simulink model "MARS"  (R2022a)
settings: Solver=VariableStepAuto  StartTime=0.0  StopTime=inf  RelTol=1e-3
model workspace (MAT data in the model file):
  T0 = -23.4
  h_trop = 7
  ingenuityParams : object (value not decoded)
symbols that are objects in the model workspace (value not decoded): ingenuityParams
undefined symbols (not defined in the file): body, collective1, collective2, duration, ingenuity, leg1, leg2, leg3, leg4, link_name, model_name, rotor1, rotor2, solarPanel, world_pose
libraries: fl_lib x35, robotgazebolib x31, nesl_utility x12, ee_lib x11, slpidlib x3, sharedtransform x2, simulink x1, shared6dof x1, aerolibwind2 x1
(part 2 of 3)

== system MARS/M.A.R.S./Force Components ==
  note: Subsystem
  In1 : Inport
  In2 : Inport  Port=2
  delta : Inport  Port=3
  epsilon : Inport  Port=4
  In5 : Inport  Port=5
  Components : Subsystem
  Product2 : Product
  Subsystem : Subsystem
  Out1 : Outport
  Out2 : Outport  Port=2
  Out3 : Outport  Port=3
  wires:
  Components/2(Out2) -> Subsystem/3(In3)
  Components/1(Out1) -> Subsystem/2(In2)
  Components/3(Out3) -> Subsystem/4(In4)
  In1/1 -> Product2/1
  Components/4(Out4) -> Subsystem/5(In5)
  Subsystem/2(Out2) -> Out2/1
  epsilon/1 -> Components/2(epsilon)
  Subsystem/1(Out1) -> Out1/1
  Product2/1 -> Subsystem/1(In1)
  Subsystem/3(Out3) -> Out3/1
  delta/1 -> Components/1(delta)
  In5/1 -> Subsystem/6(In6)
  In2/1 -> Product2/2

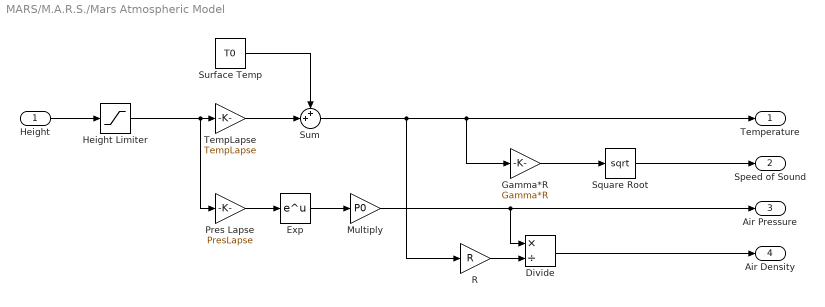
== system MARS/M.A.R.S./Mars Atmospheric Model ==
  Height : Inport
  Divide : Product  Inputs=*/
  Exp : Math
  Gamma*R : Gain  Gain=Gamma*R
  Height Limiter : Saturate  UpperLimit=height_lim  LowerLimit=0
  Multiply : Gain  Gain=P0
  Pres Lapse : Gain  Gain=PresLapse
  R : Gain  Gain=R
  Square Root : Sqrt
  Sum : Sum  Inputs=++|
  Surface Temp : Constant  Value=T0
  TempLapse : Gain  Gain=TempLapse
  Temperature : Outport  Unit=K  VectorParamsAs1DForOutWhenUnconnected=off
  Speed of Sound : Outport  Port=2  Unit=m/s  VectorParamsAs1DForOutWhenUnconnected=off
  Air Pressure : Outport  Port=3  Unit=Pa  VectorParamsAs1DForOutWhenUnconnected=off
  Air Density : Outport  Port=4  Unit=kg/m^3  VectorParamsAs1DForOutWhenUnconnected=off
  wires:
  TempLapse/1 -> Sum/2
  Surface Temp/1 -> Sum/1
  Sum/1 -> Gamma*R/1, Temperature/1, R/1
  Pres Lapse/1 -> Exp/1
  Exp/1 -> Multiply/1
  Multiply/1 -> Divide/1, Air Pressure/1
  Height/1 -> Height Limiter/1
  Height Limiter/1 -> Pres Lapse/1, TempLapse/1
  Gamma*R/1 -> Square Root/1
  Square Root/1 -> Speed of Sound/1
  R/1 -> Divide/2
  Divide/1 -> Air Density/1

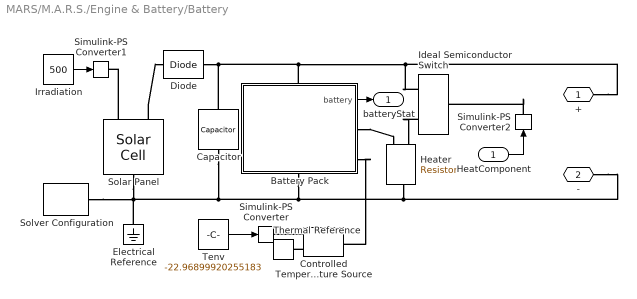
== system MARS/M.A.R.S./Engine & Battery/Battery ==
  HeatComponent : Inport
  Battery Pack : Subsystem  Variant=on  VariantControlMode=label  LabelModeActiveChoice=Detailed Battery Pack
      settings: PortSchema="{\"entries\":[{\"content\":{\"sides\":[{\"content\":{\"connectorIds\":[]},\"type\":\"ConnectorPlacement.EquallySpacedRectSide\",\"uuid\":\"b9ff85f5-5d37-4551-b274-b4f400e31e90\"},{\"content\":{\"connectorIds\":[\"Out1\",\"RConn1\",\"RConn2\"],\"side\":\"RIGHT\"},\"type\":\"ConnectorPlacement.EquallySpacedRectSide\",\"uuid\":\"9895ebaf-077a-447d-9f12-67b2d221f552\"},{\"content\":{\"connectorIds\":[\"LConn1\"],\"side\":\"TOP\"},\"type\":\"ConnectorPlacement.EquallySpacedRectSide\",\"uuid\":\"1c6b4d28-0fee-40d3-aeb3-8529f8417079\"},{\"content\":{\"connectorIds\":[\"RConn3\"],\"side\":\"BOTTOM\"},\"type\":\"ConnectorPlacement.EquallySpacedRectSide\",\"uuid\":\"bb08ee4d-4e3f-4517-9dbc-020c674c7490\"}]},\"type\":\"ConnectorPlacement.EquallySpacedConnector\",\"uuid\":\"d782096a-eb61-452d-945f-a15e6ccd7694\"}],\"packageUris\":[\"http://schema.mathworks.com/mf0/Connector/R2020b\"],\"version\":\"1.0\"}"
  Capacitor : fl_lib/Electrical/Electrical Elements/Capacitor  c=1e-6 F  r=1e-3 Ohm  g=0 1/Ohm  i_specify=off  i_priority=None  i=0 A  i_nominal_specify=off  i_nominal_unit=A  i_nominal_value=1  v_specify=off  v_priority=None  v=0 V  v_nominal_specify=off  v_nominal_unit=V  v_nominal_value=1  vc_specify=on  vc_priority=High  vc=24 V  vc_nominal_specify=off  vc_nominal_unit=V  vc_nominal_value=1
      settings: SourceProductBaseCode=PW,SS,VE  LogSimulationData=on
  Controlled Temperature Source : fl_lib/Thermal/Thermal Sources/Controlled Temperature Source
      settings: SourceProductBaseCode=PW,SS,VE
  Diode : fl_lib/Electrical/Electrical Elements/Diode  Vf=0.6 V  Ron=0.3 Ohm  Goff=1e-8 1/Ohm  i_specify=off  i_priority=None  i=0 A  i_nominal_specify=off  i_nominal_unit=A  i_nominal_value=1  v_specify=off  v_priority=None  v=0 V  v_nominal_specify=off  v_nominal_unit=V  v_nominal_value=1
      settings: SourceProductBaseCode=PW,SS,VE  LogSimulationData=on
  Electrical Reference : fl_lib/Electrical/Electrical Elements/Electrical Reference
      settings: SourceProductBaseCode=PW,SS,VE
  Heater : ee_lib/Passive/Resistor  R=2 Ohm  enable_R_tol=0  R_tol=5  tol_distribution=1  nSigma=4  enable_operating_limits=0  operating_limit_action=2  max_working_voltage=100 V  power_rating=1 W  enable_faults=0  fault_action=1  R_faulted=inf Ohm  enable_temporal_fault=0  t_fault=1 s  enable_behavioral_fault=0  max_permissible_current=1 A  t_fail_on_current=1 s  noise_mode=0  sample_time=1e-3 s  repeatability=1  auto_seed=3499211588  user_seed=0  Tdevice=25 degC  power_derating_T1=70 degC  power_derating_T2=155 degC  operating_temperature_range_vec=[-50, 150] degC  alpha=3.93e-3 1/K  Tmeas=25 degC  thermal_mass=ingenuityParams.heater.thermalMass J/K  temperature_specify=on  temperature_priority=None  temperature=ingenuityParams.battery.cell.T_init degC  temperature_nominal_specify=off  temperature_nominal_unit=K  temperature_nominal_value=1
      settings: LogSimulationData=on  InternalSimscapePortConfiguration="{\"Bottom\":[],\"Left\":[{\"id\":\"p\",\"label\":\"+\",\"type\":\"foundation.electrical.electrical\"},{\"id\":\"H\",\"label\":\"H\",\"type\":\"foundation.thermal.thermal\"}],\"Right\":[{\"id\":\"n\",\"label\":\"-\",\"type\":\"foundation.electrical.electrical\"}],\"Top\":[]}"
  Ideal Semiconductor Switch : ee_lib/Semiconductors & Converters/Ideal Semiconductor Switch  Ron=0.001 Ohm  Goff=1e-6 1/Ohm  Vth=0.5 V  diode_param=1  diode_Vf=0.8 V  diode_Ron=0.001 Ohm  diode_Goff=1e-5 1/Ohm  diode_C=50e-9 F  diode_iRM=-235 A  diode_iF=300 A  diode_idot=-50 A/us  diode_trr_param=1  diode_trr_factor=3  diode_trr=15 us  diode_Qrr=1500 s*uA
      settings: SourceProductBaseCode=PS  LogSimulationData=on
  Irradiation : Constant  Value=500
  Simulink-PS Converter : nesl_utility/Simulink-PS Converter  PhysicalDomain=network_engine_domain  SubClassName=ps_input  LeftPortType=input  RightPortType=output  PseudoPeriodic=off  Frequencies=[]  NoiseDistribution=none  NoiseParameters=[]  Unit=degC  AffineConversion=on  FilteringAndDerivatives=provide  SimscapeFilterOrder=1  InputFilterTimeConstant=0.001  UdotUserProvided=0
      settings: SourceProductBaseCode=SS,PW,VE
  Simulink-PS Converter1 : nesl_utility/Simulink-PS Converter  PhysicalDomain=network_engine_domain  SubClassName=ps_input  LeftPortType=input  RightPortType=output  PseudoPeriodic=off  Frequencies=[]  NoiseDistribution=none  NoiseParameters=[]  Unit=W/m^2  AffineConversion=off  FilteringAndDerivatives=provide  SimscapeFilterOrder=1  InputFilterTimeConstant=0.001  UdotUserProvided=0
      settings: SourceProductBaseCode=SS,PW,VE
  Simulink-PS Converter2 : nesl_utility/Simulink-PS Converter  PhysicalDomain=network_engine_domain  SubClassName=ps_input  LeftPortType=input  RightPortType=output  PseudoPeriodic=off  Frequencies=[]  NoiseDistribution=none  NoiseParameters=[]  Unit=V  AffineConversion=off  FilteringAndDerivatives=provide  SimscapeFilterOrder=1  InputFilterTimeConstant=0.001  UdotUserProvided=0
      settings: SourceProductBaseCode=SS,PW,VE
  Solar Panel : ee_lib/Sources/Solar Cell  prm=1  Isc=ingenuityParams.solarcells.Isc A  Voc=ingenuityParams.solarcells.Voc V  Is=1e-6 A  Is2=0 A  Iph=7.34 A  Ir0=ingenuityParams.solarcells.Ir0 W/m^2  ec=ingenuityParams.solarcells.qualFactor  N2=2  Rs=ingenuityParams.solarcells.Rs Ohm  Rp=inf Ohm  N_series=ingenuityParams.solarcells.Nseries  N_parallel=ingenuityParams.solarcells.Nparallel  TIPH1=0 1/K  EG=1.11 eV  TXIS1=3  TXIS2=3  TRS1=0  TRP1=0  Tmeas=25 degC  TFIXED=25 degC  thermal_mass=100 J/K  initial_temperature=25 degC
      settings: SourceProductBaseCode=PS  LogSimulationData=on
  Solver Configuration : nesl_utility/Solver Configuration  PhysicalDomain=network_engine_domain  SubClassName=solver  LeftPortType=input  RightPortType=generic  Tones=[]  Harmonics=[]  SimulateNoise=off  Profile=off  UseLocalSampling=off  EnableSwitchedLinearOptims=on  FrequencyDomain=off  UseCCode=off  RelTol=0.001  AbsTol=1e-06  MinStep=1e-09  ToWorkspace=off  RevertToSquareIcSolve=off  NumHomotopyIterations=100  PhasorMode=off  PhasorModeNumHarmonics=1  IndexReductionMethod=DerivativeReplacement  DoDC=off  ResidualTolerance=1e-09  UseLocalSolver=off  LocalSolverChoice=NE_BACKWARD_EULER_ADVANCER  LocalSolverSampleTime=0.001  DoFixedCost=off  MaxNonlinIter=3  MaxModeIter=2  ComputeImpulses=off  ImpulseIterations=2  LinearAlgebra=auto  LinearAlgebraNumThread=0  EquationFormulation=NE_TIME_EF  DelaysMemoryBudget=1024  AutomaticFiltering=on  FilteringTimeConstant=0.001  PartitionStorageMethod=AS_NEEDED  PartitionMemoryBudget=1024  PartitionMethod=ROBUST
      settings: SourceProductBaseCode=SS,PW,VE
  Tenv : Constant  Value=-22.96899920255183
  Thermal Reference : fl_lib/Thermal/Thermal Elements/Thermal Reference
      settings: SourceProductBaseCode=PW,SS,VE
  + : PMIOPort  Side=Left
  - : PMIOPort  Port=2  Side=Left
  batteryStat : Outport
  wires:
  Tenv/1 -> Simulink-PS Converter/1
  Battery Pack/1(battery) -> batteryStat/1
  HeatComponent/1 -> Simulink-PS Converter2/1
  Irradiation/1 -> Simulink-PS Converter1/1
  connections:
  Solar Panel/LConn2 -- Diode/LConn1
  Capacitor/LConn1 -- +/RConn1 -- Ideal Semiconductor Switch/RConn1 -- Battery Pack/LConn1 -- Diode/RConn1
  Controlled Temperature Source/RConn1 -- Simulink-PS Converter/RConn1
  Heater/RConn1 -- -/RConn1 -- Solver Configuration/RConn1 -- Electrical Reference/LConn1 -- Solar Panel/RConn1 -- Capacitor/RConn1 -- Battery Pack/RConn3
  Simulink-PS Converter2/RConn1 -- Ideal Semiconductor Switch/LConn1
  Ideal Semiconductor Switch/RConn2 -- Heater/LConn1
  Controlled Temperature Source/RConn2 -- Thermal Reference/LConn1
  Solar Panel/LConn1 -- Simulink-PS Converter1/RConn1
  Battery Pack/RConn2 -- Controlled Temperature Source/LConn1
  Battery Pack/RConn1 -- Heater/LConn2

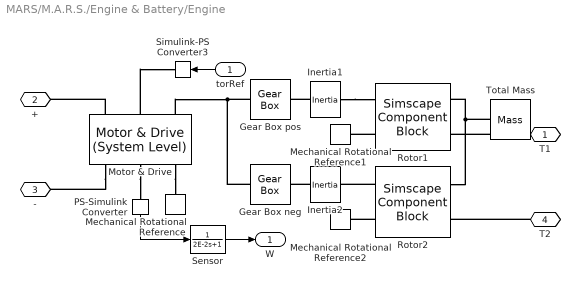
== system MARS/M.A.R.S./Engine & Battery/Engine ==
  torRef : Inport
  Gear Box neg : fl_lib/Mechanical/Mechanisms/Gear Box  ratio=-1*ingenuityParams.gearbox.ratio  t_in_specify=off  t_in_priority=None  t_in=0 N*m  t_in_nominal_specify=off  t_in_nominal_unit=N*m  t_in_nominal_value=1  t_out_specify=off  t_out_priority=None  t_out=0 N*m  t_out_nominal_specify=off  t_out_nominal_unit=N*m  t_out_nominal_value=1
      settings: SourceProductBaseCode=PW,SS,VE  LogSimulationData=on
  Gear Box pos : fl_lib/Mechanical/Mechanisms/Gear Box  ratio=ingenuityParams.gearbox.ratio  t_in_specify=off  t_in_priority=None  t_in=0 N*m  t_in_nominal_specify=off  t_in_nominal_unit=N*m  t_in_nominal_value=1  t_out_specify=off  t_out_priority=None  t_out=0 N*m  t_out_nominal_specify=off  t_out_nominal_unit=N*m  t_out_nominal_value=1
      settings: SourceProductBaseCode=PW,SS,VE  LogSimulationData=on
  Inertia1 : fl_lib/Mechanical/Rotational Elements/Inertia  inertia=ingenuityParams.propeller.inertia kg*m^2  num_ports=foundation.enum.numPorts2.two  w_specify=off  w_priority=High  w=0 rad/s  w_nominal_specify=off  w_nominal_unit=rad/s  w_nominal_value=1  t_specify=off  t_priority=None  t=0 N*m  t_nominal_specify=off  t_nominal_unit=N*m  t_nominal_value=1
      settings: SourceProductBaseCode=PW,SS,VE  LogSimulationData=on  InternalSimscapePortConfiguration="{\"Bottom\":[],\"Left\":[{\"id\":\"I\",\"label\":\"\",\"type\":\"foundation.mechanical.rotational.rotational\"}],\"Right\":[{\"id\":\"J\",\"label\":\"\",\"type\":\"foundation.mechanical.rotational.rotational\"}],\"Top\":[]}"
  Inertia2 : fl_lib/Mechanical/Rotational Elements/Inertia  inertia=ingenuityParams.propeller.inertia kg*m^2  num_ports=foundation.enum.numPorts2.two  w_specify=off  w_priority=High  w=0 rad/s  w_nominal_specify=off  w_nominal_unit=rad/s  w_nominal_value=1  t_specify=off  t_priority=None  t=0 N*m  t_nominal_specify=off  t_nominal_unit=N*m  t_nominal_value=1
      settings: SourceProductBaseCode=PW,SS,VE  LogSimulationData=on  InternalSimscapePortConfiguration="{\"Bottom\":[],\"Left\":[{\"id\":\"I\",\"label\":\"\",\"type\":\"foundation.mechanical.rotational.rotational\"}],\"Right\":[{\"id\":\"J\",\"label\":\"\",\"type\":\"foundation.mechanical.rotational.rotational\"}],\"Top\":[]}"
  Mechanical Rotational Reference : fl_lib/Mechanical/Rotational Elements/Mechanical Rotational Reference
      settings: SourceProductBaseCode=PW,SS,VE
  Mechanical Rotational Reference1 : fl_lib/Mechanical/Rotational Elements/Mechanical Rotational Reference
      settings: SourceProductBaseCode=PW,SS,VE
  Mechanical Rotational Reference2 : fl_lib/Mechanical/Rotational Elements/Mechanical Rotational Reference
      settings: SourceProductBaseCode=PW,SS,VE
  Motor & Drive : ee_lib/Electromechanical/Motor & Drive (System Level)  torque_speed_param=ee.enum.electromech.envelope.torque_power  overtorque_param=ee.enum.electromech.overtorque.no  T_t=[.09, .08, .07, 0] N*m  T_t_intermittent=[.36, .32, .28, 0] N*m  T_t_2D=[.09, .09, .09; .08, .08, .08; .07, .07, .07; 0, 0, 0] N*m  T_t_intermittent_2D=[.36, .36, .36; .32, .32, .32; .28, .28, .28; 0, 0, 0] N*m  w_t=[0, 3750, 7500, 8000] rpm  vdc_t=[6, 12, 24] V  torque_max=ingenuityParams.motordrive.torMax N*m  power_max=ingenuityParams.motordrive.powMax W  torque_max_intermittent=0.4 N*m  power_max_intermittent=120 W  time_overtorque=30 s  time_recover=60 s  Tc=ingenuityParams.motordrive.Tc s  losses_param=1  eff=ingenuityParams.motordrive.effRated  w_eff=ingenuityParams.motordrive.wRated rpm  T_eff=ingenuityParams.motordrive.torRated N*m  Piron=ingenuityParams.motordrive.ironLoss W  Pbase=ingenuityParams.motordrive.fixedLoss W  w_eff_vec=[-8000, -4000, 0, 4000, 8000] rpm  T_eff_vec=[0, .03, .06, .09] N*m  v_eff_vec=[100, 250, 400] V  losses_mat=[1.49, 1.67, 2.21, 3.1; .42, .69, 1.14, 2.03; .06, .24, .78, 1.68; .42, .69, 1.14, 2.03; 1.49, 1.67, 2.21, 3.1] W  efficiency_mat=[95, 95, 95, 95; 95, 95, 95, 95; 95, 95, 95, 95; 95, 95, 95, 95; 95, 95, 95, 95]  losses_mat_3D=ones(5, 4, 3) W  efficiency_mat_3D=95 * ones(5, 4, 3)  Res=ingenuityParams.motordrive.supplyRes Ohm  enable_fault=simscape.enum.onoff.off  fault_condition=1  fault_threshold=0.5  J=0 kg*m^2  lam=0 N*m/(rad/s)  speed0=0 rpm  faulted_specify=off  faulted_priority=None  faulted=0  faulted_nominal_specify=off  faulted_nominal_unit=1  faulted_nominal_value=1  torqueLimitContinuous_specify=off  torqueLimitContinuous_priority=None  torqueLimitContinuous=0 N*m  torqueLimitContinuous_nominal_specify=off  torqueLimitContinuous_nominal_unit=N*m  torqueLimitContinuous_nominal_value=1  alpha=3.93e-3 1/K  Tmeas=25 degC  Tmeas2=125 degC  losses_mat_T2=[1.49, 1.74, 2.49, 3.74; .42, .67, 1.42, 2.67; .06, .31, 1.06, 2.31; .42, .67, 1.42, 2.67; 1.49, 1.74, 2.49, 3.74] W  efficiency_mat_T2=[95, 95, 95, 95; 95, 95, 95, 95; 95, 95, 95, 95; 95, 95, 95, 95; 95, 95, 95, 95]  losses_mat_3D_T2=ones(5, 4, 3) W  efficiency_mat_3D_T2=95 * ones(5, 4, 3)  thermal_mass=100 J/K  initial_temperature=25 degC
      settings: SourceProductBaseCode=PS  LogSimulationData=on
  PS-Simulink Converter : nesl_utility/PS-Simulink Converter  PhysicalDomain=network_engine_domain  SubClassName=ps_output  LeftPortType=input  RightPortType=output  PseudoPeriodic=off  Frequencies=[]  VectorFormat=1-D array  Unit=rad/s  AffineConversion=off
      settings: SourceProductBaseCode=SS,PW,VE
  Rotor1 : SimscapeComponentBlock  SourceFile=simple_rotor  ComponentPath=simple_rotor  ComponentVariants="[\"simple_rotor\"]"  ComponentVariantNames="[\"simple_rotor\"]"  ClassName=simple_rotor  SchemaVersion=1  rot_dir=simscape.enum.posneg.positive  D=ingenuityParams.propeller.diameter m  J_TLU=ingenuityParams.propeller.Jvec  k_thrust_TLU=ingenuityParams.propeller.kTvec  k_power_TLU=ingenuityParams.propeller.kPvec  interp_method=simscape.enum.interpolation.smooth  extrap_method=simscape.enum.extrapolation.linear  density=ingenuityParams.environment.atmDensity kg/m^3  n_thr=1e-2 Hz  w_specify=on  w_priority=None  w=0 rpm  w_nominal_specify=off  w_nominal_unit=rad/s  w_nominal_value=1  Q_specify=off  Q_priority=None  Q=0 N*m  Q_nominal_specify=off  Q_nominal_unit=N*m  Q_nominal_value=1
      settings: CopyFcn=simscape.engine.sli.internal.componentblockcallback(gcbh,'COPY')  PreCopyFcn=simscape.engine.sli.internal.componentblockcallback(gcbh,'PRECOPY')  PreDeleteFcn=simscape.engine.sli.internal.componentblockcallback(gcbh,'PREDELETE')  InternalSimscapePortConfiguration="{\"Bottom\":[],\"Left\":[{\"id\":\"R\",\"label\":\"R\",\"type\":\"foundation.mechanical.rotational.rotational\"},{\"id\":\"C\",\"label\":\"C\",\"type\":\"foundation.mechanical.rotational.rotational\"}],\"Right\":[{\"id\":\"V\",\"label\":\"V\",\"type\":\"foundation.mechanical.translational.translational\"},{\"id\":\"T\",\"label\":\"T\",\"type\":\"output\"}],\"Top\":[]}"
      mask Type: Simple Rotor
  Rotor2 : SimscapeComponentBlock  SourceFile=simple_rotor  ComponentPath=simple_rotor  ComponentVariants="[\"simple_rotor\"]"  ComponentVariantNames="[\"simple_rotor\"]"  ClassName=simple_rotor  SchemaVersion=1  rot_dir=simscape.enum.posneg.positive  D=ingenuityParams.propeller.diameter m  J_TLU=ingenuityParams.propeller.Jvec  k_thrust_TLU=ingenuityParams.propeller.kTvec  k_power_TLU=ingenuityParams.propeller.kPvec  interp_method=simscape.enum.interpolation.smooth  extrap_method=simscape.enum.extrapolation.linear  density=ingenuityParams.environment.atmDensity kg/m^3  n_thr=1e-2 Hz  w_specify=on  w_priority=None  w=0 rpm  w_nominal_specify=off  w_nominal_unit=rad/s  w_nominal_value=1  Q_specify=off  Q_priority=None  Q=0 N*m  Q_nominal_specify=off  Q_nominal_unit=N*m  Q_nominal_value=1
      settings: CopyFcn=simscape.engine.sli.internal.componentblockcallback(gcbh,'COPY')  PreCopyFcn=simscape.engine.sli.internal.componentblockcallback(gcbh,'PRECOPY')  PreDeleteFcn=simscape.engine.sli.internal.componentblockcallback(gcbh,'PREDELETE')  InternalSimscapePortConfiguration="{\"Bottom\":[],\"Left\":[{\"id\":\"R\",\"label\":\"R\",\"type\":\"foundation.mechanical.rotational.rotational\"},{\"id\":\"C\",\"label\":\"C\",\"type\":\"foundation.mechanical.rotational.rotational\"}],\"Right\":[{\"id\":\"V\",\"label\":\"V\",\"type\":\"foundation.mechanical.translational.translational\"},{\"id\":\"T\",\"label\":\"T\",\"type\":\"output\"}],\"Top\":[]}"
      mask Type: Simple Rotor
  Sensor : TransferFcn  Denominator=[2E-2 1]
  Simulink-PS Converter3 : nesl_utility/Simulink-PS Converter  PhysicalDomain=network_engine_domain  SubClassName=ps_input  LeftPortType=input  RightPortType=output  PseudoPeriodic=off  Frequencies=[]  NoiseDistribution=none  NoiseParameters=[]  Unit=N*m  AffineConversion=off  FilteringAndDerivatives=provide  SimscapeFilterOrder=1  InputFilterTimeConstant=0.001  UdotUserProvided=0
      settings: SourceProductBaseCode=SS,PW,VE
  Total Mass : fl_lib/Mechanical/Translational Elements/Mass  mass=ingenuityParams.mechanical.totalMassExceptBatteries + ingenuityParams.battery.numCells*ingenuityParams.battery.cell.mass kg  num_ports=foundation.enum.numPorts2.one  v_specify=off  v_priority=High  v=0 m/s  v_nominal_specify=off  v_nominal_unit=m/s  v_nominal_value=1  f_specify=off  f_priority=None  f=0 N  f_nominal_specify=off  f_nominal_unit=N  f_nominal_value=1
      settings: SourceProductBaseCode=PW,SS,VE  LogSimulationData=on
  T1 : PMIOPort  Side=Right
  + : PMIOPort  Port=2  Side=Left
  - : PMIOPort  Port=3  Side=Left
  T2 : PMIOPort  Port=4  Side=Right
  W : Outport
  wires:
  torRef/1 -> Simulink-PS Converter3/1
  Sensor/1 -> W/1
  PS-Simulink Converter/1 -> Sensor/1
  connections:
  Inertia1/RConn1 -- Gear Box pos/RConn1
  Inertia2/RConn1 -- Gear Box neg/RConn1
  T1/RConn1 -- Rotor1/RConn2
  Inertia1/LConn1 -- Rotor1/LConn1
  Motor & Drive/LConn1 -- +/RConn1
  Rotor1/LConn2 -- Mechanical Rotational Reference1/LConn1
  Motor & Drive/RConn2 -- PS-Simulink Converter/LConn1
  Motor & Drive/LConn2 -- Simulink-PS Converter3/RConn1
  T2/RConn1 -- Rotor2/RConn2
  Gear Box pos/LConn1 -- Motor & Drive/LConn3 -- Gear Box neg/LConn1
  Motor & Drive/RConn1 -- -/RConn1
  Motor & Drive/RConn3 -- Mechanical Rotational Reference/LConn1
  Rotor2/LConn1 -- Inertia2/LConn1
  Total Mass/LConn1 -- Rotor2/RConn1 -- Rotor1/RConn1
  Rotor2/LConn2 -- Mechanical Rotational Reference2/LConn1

== system MARS/M.A.R.S./Force Components/Components ==
  delta : Inport
  epsilon : Inport  Port=2
  Cos : Trigonometry  Operator=cos
  Cos1 : Trigonometry  Operator=cos
  Sin : Trigonometry
  Sin1 : Trigonometry
  Out1 : Outport
  Out2 : Outport  Port=2
  Out3 : Outport  Port=3
  Out4 : Outport  Port=4
  wires:
  delta/1 -> Cos/1, Sin/1
  Sin1/1 -> Out4/1
  Cos/1 -> Out1/1
  Cos1/1 -> Out2/1
  Sin/1 -> Out3/1
  epsilon/1 -> Cos1/1, Sin1/1

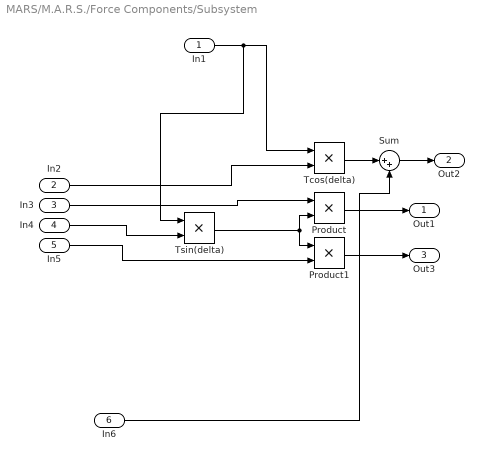
== system MARS/M.A.R.S./Force Components/Subsystem ==
  In1 : Inport
  In2 : Inport  Port=2
  In3 : Inport  Port=3
  In4 : Inport  Port=4
  In5 : Inport  Port=5
  In6 : Inport  Port=6
  Product : Product
  Product1 : Product
  Sum : Sum  Inputs=|++
  Tcos(delta) : Product
  Tsin(delta) : Product
  Out1 : Outport
  Out2 : Outport  Port=2
  Out3 : Outport  Port=3
  wires:
  In6/1 -> Sum/2
  Product1/1 -> Out3/1
  In1/1 -> Tsin(delta)/1, Tcos(delta)/1
  Tsin(delta)/1 -> Product/2, Product1/1
  In4/1 -> Tsin(delta)/2
  Tcos(delta)/1 -> Sum/1
  In5/1 -> Product1/2
  Product/1 -> Out1/1
  In2/1 -> Tcos(delta)/2
  In3/1 -> Product/1
  Sum/1 -> Out2/1

== system MARS/M.A.R.S./Engine & Battery/Battery/Battery Pack ==
  Detailed Battery Pack : Subsystem  VariantControl=Detailed Battery Pack
      settings: PortSchema="{\"entries\":[{\"content\":{\"sides\":[{\"content\":{\"connectorIds\":[]},\"type\":\"ConnectorPlacement.EquallySpacedRectSide\",\"uuid\":\"ac491242-3df9-473d-beed-1a2139a6c6bd\"},{\"content\":{\"connectorIds\":[\"Out1\",\"RConn1\",\"RConn2\"],\"side\":\"RIGHT\"},\"type\":\"ConnectorPlacement.EquallySpacedRectSide\",\"uuid\":\"5d11d2aa-1dd1-475e-9911-89b4672a4360\"},{\"content\":{\"connectorIds\":[\"LConn1\"],\"side\":\"TOP\"},\"type\":\"ConnectorPlacement.EquallySpacedRectSide\",\"uuid\":\"d9fa746a-c212-49ba-8905-bd0b35a53459\"},{\"content\":{\"connectorIds\":[\"RConn3\"],\"side\":\"BOTTOM\"},\"type\":\"ConnectorPlacement.EquallySpacedRectSide\",\"uuid\":\"9203f755-4900-467a-80ce-d49a17dbef8c\"}]},\"type\":\"ConnectorPlacement.EquallySpacedConnector\",\"uuid\":\"8e24b369-26fe-4156-84c2-0f7c31bd4a1a\"}],\"packageUris\":[\"http://schema.mathworks.com/mf0/Connector/R2020b\"],\"version\":\"1.0\"}"
  Simplified Battery Pack : Subsystem  VariantControl=Simplified Battery Pack
      settings: PortSchema="{\"entries\":[{\"content\":{\"sides\":[{\"content\":{\"connectorIds\":[]},\"type\":\"ConnectorPlacement.EquallySpacedRectSide\",\"uuid\":\"ac491242-3df9-473d-beed-1a2139a6c6bd\"},{\"content\":{\"connectorIds\":[\"Out1\",\"RConn1\",\"RConn2\"],\"side\":\"RIGHT\"},\"type\":\"ConnectorPlacement.EquallySpacedRectSide\",\"uuid\":\"5d11d2aa-1dd1-475e-9911-89b4672a4360\"},{\"content\":{\"connectorIds\":[\"LConn1\"],\"side\":\"TOP\"},\"type\":\"ConnectorPlacement.EquallySpacedRectSide\",\"uuid\":\"d9fa746a-c212-49ba-8905-bd0b35a53459\"},{\"content\":{\"connectorIds\":[\"RConn3\"],\"side\":\"BOTTOM\"},\"type\":\"ConnectorPlacement.EquallySpacedRectSide\",\"uuid\":\"ceef3f59-c6c2-4ed7-8bde-a1c8d7ba1997\"}]},\"type\":\"ConnectorPlacement.EquallySpacedConnector\",\"uuid\":\"8e24b369-26fe-4156-84c2-0f7c31bd4a1a\"}],\"packageUris\":[\"http://schema.mathworks.com/mf0/Connector/R2020b\"],\"version\":\"1.0\"}"
  + : PMIOPort  Side=Left
  HEAT : PMIOPort  Port=2  Side=Right
  ENV : PMIOPort  Port=3  Side=Right
  - : PMIOPort  Port=4  Side=Right
  battery : Outport

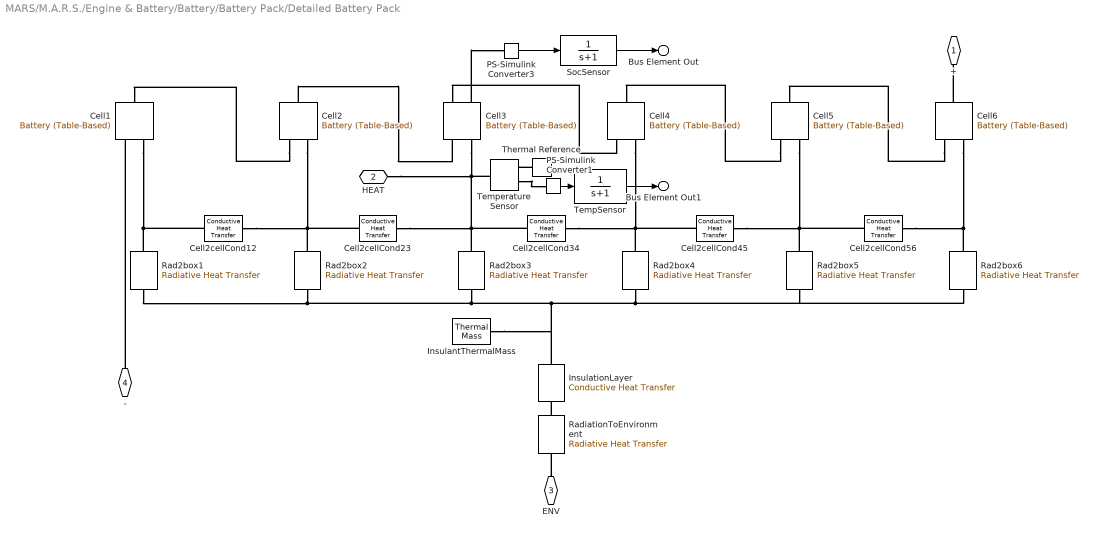
== system MARS/M.A.R.S./Engine & Battery/Battery/Battery Pack/Detailed Battery Pack ==
  Cell{1..2,4..6} (5 alike) : ee_lib/Sources/Battery (Table-Based)  SOC_vec=ingenuityParams.battery.cell.SOCvec  T_dependence=ee.enum.temperature_dependence.yes  prm_dir=ee.enum.battery.prm_dir.noCurrentDirectionality  T_vec=ingenuityParams.battery.cell.Tvec degC  V0_mat=ingenuityParams.battery.cell.V0_TLU V  V0_vec=[3.1, 3.27, 3.31, 3.5] V  R0_mat=ingenuityParams.battery.cell.R0_TLU Ohm  R0_vec=[.015, .017, .012, .013] Ohm  R0_dis_mat=[.03, .015, .002; .04, .017, .008; .039, .012, .006; .027, .013, .021] Ohm  R0_dis_vec=[.015, .017, .012, .013] Ohm  R0_ch_mat=[.03, .015, .002; .04, .017, .008; .039, .012, .006; .027, .013, .021] Ohm  R0_ch_vec=[.015, .017, .012, .013] Ohm  AH=ingenuityParams.battery.cell.AH_TLU hr*A  prm_leak=ee.enum.battery.prm_leak.disabled  Rleak_vec=[8000, 7000, 6000] Ohm  Rleak=7e3 Ohm  extrapolation_option=simscape.enum.extrapolation.nearest  SOC_port=ee.enum.enable.no  V_range=[0, inf] V  prm_dyn=ee.enum.battery.prm_dyn.off  R1_mat=[.089, .076, .01; .042, .022, .099; .019, .007, .002; .051, .043, .029] Ohm  R1_vec=[.076, .022, .007, .043] Ohm  tau1_mat=[44, 148, 235; 93, 110, 1000; 19, 27, 133; .5, 22, 3] s  tau1_vec=[148, 110, 27, 22] s  R2_mat=[.014, .382, .407; .028, .006, .007; .014, .007, .006; .333, .956, .912] Ohm  R2_vec=[.382, .006, .007, .956] Ohm  tau2_mat=[1, 44, 5644; 11, 24, 506; 2, 14, 330; 3310, 13419, 30216] s  tau2_vec=[44, 24, 14, 13419] s  R3_mat=[.014, .382, .407; .028, .006, .007; .014, .007, .006; .333, .956, .912] Ohm  R3_vec=[.382, .006, .007, .956] Ohm  tau3_mat=[1, 44, 5644; 11, 24, 506; 2, 14, 330; 3310, 13419, 30216] s  tau3_vec=[44, 24, 14, 13419] s  R4_mat=[.014, .382, .407; .028, .006, .007; .014, .007, .006; .333, .956, .912] Ohm  R4_vec=[.382, .006, .007, .956] Ohm  tau4_mat=[1, 44, 5644; 11, 24, 506; 2, 14, 330; 3310, 13419, 30216] s  tau4_vec=[44, 24, 14, 13419] s  R5_mat=[.014, .382, .407; .028, .006, .007; .014, .007, .006; .333, .956, .912] Ohm  R5_vec=[.382, .006, .007, .956] Ohm  tau5_mat=[1, 44, 5644; 11, 24, 506; 2, 14, 330; 3310, 13419, 30216] s  tau5_vec=[44, 24, 14, 13419] s  prm_fade=ee.enum.battery.prm_fade.equations  N0=100  dV0=0  dR0=0  dAH=0  dRleak=0  dR1=0  dR2=0  dR3=0  dR4=0  dR5=0  N0vec=[100, 200, 300]  Tfadevec=[298.15, 323.15] K  dV0vec=[0, 0, 0]  dR0vec=[0, 0, 0]  dAHvec=[0, 0, 0]  dRleakvec=[0, 0, 0]  dR1vec=[0, 0, 0]  dR2vec=[0, 0, 0]  dR3vec=[0, 0, 0]  dR4vec=[0, 0, 0]  dR5vec=[0, 0, 0]  dV0mat=[0, 0; 0, 0; 0, 0]  dR0mat=[0, 0; 0, 0; 0, 0]  dAHmat=[0, 0; 0, 0; 0, 0]  dRleakmat=[0, 0; 0, 0; 0, 0]  dR1mat=[0, 0; 0, 0; 0, 0]  dR2mat=[0, 0; 0, 0; 0, 0]  dR3mat=[0, 0; 0, 0; 0, 0]  dR4mat=[0, 0; 0, 0; 0, 0]  dR5mat=[0, 0; 0, 0; 0, 0]  prm_age_modeling=ee.enum.battery.prm_age_modeling.equation  storage_dt_age_vec=[0] d  storage_T_age_vec=[273] K  prm_age_OCV=ee.enum.battery.prm_age_OCV.OCV  OCV_age=0.9  SOC_age=0.6  prm_age_resistance=ee.enum.battery.prm_age.disabled  OCV_scaling_age_resistance=2.2134e6  OCV_offset_age_resistance=1.632e6  temp_exp_age_resistance=0.515833569 V  t_exp_age_resistance=0.75  T_age_vec_resistance=[273.15, 298.15, 323.15] K  dt_age_vec_resistance=[90, 180, 270, 360] d  dR0_age_vec=[0, 0, 0]  t_meas_dR0_age=100 d  dR0_age_mat=[0, 0, 0; 0, 0, 0; 0, 0, 0; 0, 0, 0]  prm_age_capacity=ee.enum.battery.prm_age.disabled  OCV_scaling_age_capacity=1.5097e07  OCV_offset_age_capacity=8.3625e06  temp_exp_age_capacity=0.6011 V  t_exp_age_capacity=0.75  T_age_vec_capacity=[273.15, 298.15, 323.15] K  dt_age_vec_capacity=[90, 180, 270, 360] d  dAH_age_vec=[0, 0, 0]  t_meas_dAH_age=100 d  dAH_age_mat=[0, 0, 0; 0, 0, 0; 0, 0, 0; 0, 0, 0]  thermal_port=simscape.enum.thermaleffects.model  temperature=ingenuityParams.battery.cell.T_init degC  thermal_mass=ingenuityParams.battery.cell.mass*ingenuityParams.battery.cell.cp J/K  i_specify=off  i_priority=None  i=0 A  i_nominal_specify=off  i_nominal_unit=A  i_nominal_value=1  v_specify=off  v_priority=None  v=0 V  v_nominal_specify=off  v_nominal_unit=V  v_nominal_value=1  stateOfCharge_specify=on  stateOfCharge_priority=High  stateOfCharge=ingenuityParams.battery.cell.SOC_init  stateOfCharge_nominal_specify=off  stateOfCharge_nominal_unit=1  stateOfCharge_nominal_value=1  num_cycles_specify=off  num_cycles_priority=High  num_cycles=0  num_cycles_nominal_specify=off  num_cycles_nominal_unit=1  num_cycles_nominal_value=1  cell_temperature_specify=on  cell_temperature_priority=High  cell_temperature=ingenuityParams.battery.cell.T_init degC  cell_temperature_nominal_specify=off  cell_temperature_nominal_unit=K  cell_temperature_nominal_value=1
      settings: SourceProductBaseCode=PS  LogSimulationData=on  InternalSimscapePortConfiguration="{\"Bottom\":[],\"Left\":[{\"id\":\"p\",\"label\":\"+\",\"type\":\"foundation.electrical.electrical\"}],\"Right\":[{\"id\":\"n\",\"label\":\"-\",\"type\":\"foundation.electrical.electrical\"},{\"id\":\"H\",\"label\":\"H\",\"type\":\"foundation.thermal.thermal\"}],\"Top\":[]}"
  Cell2cellCond{12,23,34,45,56} (5 alike) : fl_lib/Thermal/Thermal Elements/Conductive Heat Transfer  area=ingenuityParams.battery.thermal.cell2cellCond.area m^2  thickness=ingenuityParams.battery.thermal.cell2cellCond.thick m  th_cond=ingenuityParams.battery.thermal.cell2cellCond.k W/(m*K)  T_specify=off  T_priority=None  T=0 K  T_nominal_specify=off  T_nominal_unit=K  T_nominal_value=1  Q_specify=off  Q_priority=None  Q=0 W  Q_nominal_specify=off  Q_nominal_unit=W  Q_nominal_value=1
      settings: SourceProductBaseCode=PW,SS,VE  LogSimulationData=on
  Cell3 : ee_lib/Sources/Battery (Table-Based)  SOC_vec=ingenuityParams.battery.cell.SOCvec  T_dependence=ee.enum.temperature_dependence.yes  prm_dir=ee.enum.battery.prm_dir.noCurrentDirectionality  T_vec=ingenuityParams.battery.cell.Tvec degC  V0_mat=ingenuityParams.battery.cell.V0_TLU V  V0_vec=[3.1, 3.27, 3.31, 3.5] V  R0_mat=ingenuityParams.battery.cell.R0_TLU Ohm  R0_vec=[.015, .017, .012, .013] Ohm  R0_dis_mat=[.03, .015, .002; .04, .017, .008; .039, .012, .006; .027, .013, .021] Ohm  R0_dis_vec=[.015, .017, .012, .013] Ohm  R0_ch_mat=[.03, .015, .002; .04, .017, .008; .039, .012, .006; .027, .013, .021] Ohm  R0_ch_vec=[.015, .017, .012, .013] Ohm  AH=ingenuityParams.battery.cell.AH_TLU hr*A  prm_leak=ee.enum.battery.prm_leak.disabled  Rleak_vec=[8000, 7000, 6000] Ohm  Rleak=7e3 Ohm  extrapolation_option=simscape.enum.extrapolation.nearest  SOC_port=ee.enum.enable.yes  V_range=[0, inf] V  prm_dyn=ee.enum.battery.prm_dyn.off  R1_mat=[.089, .076, .01; .042, .022, .099; .019, .007, .002; .051, .043, .029] Ohm  R1_vec=[.076, .022, .007, .043] Ohm  tau1_mat=[44, 148, 235; 93, 110, 1000; 19, 27, 133; .5, 22, 3] s  tau1_vec=[148, 110, 27, 22] s  R2_mat=[.014, .382, .407; .028, .006, .007; .014, .007, .006; .333, .956, .912] Ohm  R2_vec=[.382, .006, .007, .956] Ohm  tau2_mat=[1, 44, 5644; 11, 24, 506; 2, 14, 330; 3310, 13419, 30216] s  tau2_vec=[44, 24, 14, 13419] s  R3_mat=[.014, .382, .407; .028, .006, .007; .014, .007, .006; .333, .956, .912] Ohm  R3_vec=[.382, .006, .007, .956] Ohm  tau3_mat=[1, 44, 5644; 11, 24, 506; 2, 14, 330; 3310, 13419, 30216] s  tau3_vec=[44, 24, 14, 13419] s  R4_mat=[.014, .382, .407; .028, .006, .007; .014, .007, .006; .333, .956, .912] Ohm  R4_vec=[.382, .006, .007, .956] Ohm  tau4_mat=[1, 44, 5644; 11, 24, 506; 2, 14, 330; 3310, 13419, 30216] s  tau4_vec=[44, 24, 14, 13419] s  R5_mat=[.014, .382, .407; .028, .006, .007; .014, .007, .006; .333, .956, .912] Ohm  R5_vec=[.382, .006, .007, .956] Ohm  tau5_mat=[1, 44, 5644; 11, 24, 506; 2, 14, 330; 3310, 13419, 30216] s  tau5_vec=[44, 24, 14, 13419] s  prm_fade=ee.enum.battery.prm_fade.equations  N0=100  dV0=0  dR0=0  dAH=0  dRleak=0  dR1=0  dR2=0  dR3=0  dR4=0  dR5=0  N0vec=[100, 200, 300]  Tfadevec=[298.15, 323.15] K  dV0vec=[0, 0, 0]  dR0vec=[0, 0, 0]  dAHvec=[0, 0, 0]  dRleakvec=[0, 0, 0]  dR1vec=[0, 0, 0]  dR2vec=[0, 0, 0]  dR3vec=[0, 0, 0]  dR4vec=[0, 0, 0]  dR5vec=[0, 0, 0]  dV0mat=[0, 0; 0, 0; 0, 0]  dR0mat=[0, 0; 0, 0; 0, 0]  dAHmat=[0, 0; 0, 0; 0, 0]  dRleakmat=[0, 0; 0, 0; 0, 0]  dR1mat=[0, 0; 0, 0; 0, 0]  dR2mat=[0, 0; 0, 0; 0, 0]  dR3mat=[0, 0; 0, 0; 0, 0]  dR4mat=[0, 0; 0, 0; 0, 0]  dR5mat=[0, 0; 0, 0; 0, 0]  prm_age_modeling=ee.enum.battery.prm_age_modeling.equation  storage_dt_age_vec=[0] d  storage_T_age_vec=[273] K  prm_age_OCV=ee.enum.battery.prm_age_OCV.OCV  OCV_age=0.9  SOC_age=0.6  prm_age_resistance=ee.enum.battery.prm_age.disabled  OCV_scaling_age_resistance=2.2134e6  OCV_offset_age_resistance=1.632e6  temp_exp_age_resistance=0.515833569 V  t_exp_age_resistance=0.75  T_age_vec_resistance=[273.15, 298.15, 323.15] K  dt_age_vec_resistance=[90, 180, 270, 360] d  dR0_age_vec=[0, 0, 0]  t_meas_dR0_age=100 d  dR0_age_mat=[0, 0, 0; 0, 0, 0; 0, 0, 0; 0, 0, 0]  prm_age_capacity=ee.enum.battery.prm_age.disabled  OCV_scaling_age_capacity=1.5097e07  OCV_offset_age_capacity=8.3625e06  temp_exp_age_capacity=0.6011 V  t_exp_age_capacity=0.75  T_age_vec_capacity=[273.15, 298.15, 323.15] K  dt_age_vec_capacity=[90, 180, 270, 360] d  dAH_age_vec=[0, 0, 0]  t_meas_dAH_age=100 d  dAH_age_mat=[0, 0, 0; 0, 0, 0; 0, 0, 0; 0, 0, 0]  thermal_port=simscape.enum.thermaleffects.model  temperature=ingenuityParams.battery.cell.T_init degC  thermal_mass=ingenuityParams.battery.cell.mass*ingenuityParams.battery.cell.cp J/K  i_specify=off  i_priority=None  i=0 A  i_nominal_specify=off  i_nominal_unit=A  i_nominal_value=1  v_specify=off  v_priority=None  v=0 V  v_nominal_specify=off  v_nominal_unit=V  v_nominal_value=1  stateOfCharge_specify=on  stateOfCharge_priority=High  stateOfCharge=ingenuityParams.battery.cell.SOC_init  stateOfCharge_nominal_specify=off  stateOfCharge_nominal_unit=1  stateOfCharge_nominal_value=1  num_cycles_specify=off  num_cycles_priority=High  num_cycles=0  num_cycles_nominal_specify=off  num_cycles_nominal_unit=1  num_cycles_nominal_value=1  cell_temperature_specify=on  cell_temperature_priority=High  cell_temperature=ingenuityParams.battery.cell.T_init degC  cell_temperature_nominal_specify=off  cell_temperature_nominal_unit=K  cell_temperature_nominal_value=1
      settings: SourceProductBaseCode=PS  LogSimulationData=on  InternalSimscapePortConfiguration="{\"Bottom\":[],\"Left\":[{\"id\":\"p\",\"label\":\"+\",\"type\":\"foundation.electrical.electrical\"},{\"id\":\"soc\",\"label\":\"SOC\",\"type\":\"output\"}],\"Right\":[{\"id\":\"n\",\"label\":\"-\",\"type\":\"foundation.electrical.electrical\"},{\"id\":\"H\",\"label\":\"H\",\"type\":\"foundation.thermal.thermal\"}],\"Top\":[]}"
  InsulantThermalMass : fl_lib/Thermal/Thermal Elements/Thermal Mass  mass=ingenuityParams.battery.thermal.insulantThermalMass.mass kg  sp_heat=ingenuityParams.battery.thermal.insulantThermalMass.cp J/kg/K  T_specify=on  T_priority=High  T=ingenuityParams.battery.cell.T_init degC  T_nominal_specify=off  T_nominal_unit=K  T_nominal_value=1  Q_specify=off  Q_priority=None  Q=0 W  Q_nominal_specify=off  Q_nominal_unit=W  Q_nominal_value=1
      settings: SourceProductBaseCode=PW,SS,VE  LogSimulationData=on
  InsulationLayer : fl_lib/Thermal/Thermal Elements/Conductive Heat Transfer  area=ingenuityParams.battery.thermal.insulationLayer.area m^2  thickness=ingenuityParams.battery.thermal.insulationLayer.thick m  th_cond=ingenuityParams.battery.thermal.insulationLayer.k W/(m*K)  T_specify=off  T_priority=None  T=0 K  T_nominal_specify=off  T_nominal_unit=K  T_nominal_value=1  Q_specify=off  Q_priority=None  Q=0 W  Q_nominal_specify=off  Q_nominal_unit=W  Q_nominal_value=1
      settings: SourceProductBaseCode=PW,SS,VE  LogSimulationData=on
  PS-Simulink Converter1 : nesl_utility/PS-Simulink Converter  PhysicalDomain=network_engine_domain  SubClassName=ps_output  LeftPortType=input  RightPortType=output  PseudoPeriodic=off  Frequencies=[]  VectorFormat=1-D array  Unit=degC  AffineConversion=on
      settings: SourceProductBaseCode=SS,PW,VE
  PS-Simulink Converter3 : nesl_utility/PS-Simulink Converter  PhysicalDomain=network_engine_domain  SubClassName=ps_output  LeftPortType=input  RightPortType=output  PseudoPeriodic=off  Frequencies=[]  VectorFormat=1-D array  Unit=1  AffineConversion=off
      settings: SourceProductBaseCode=SS,PW,VE
  Rad2box{1..6} (6 alike) : fl_lib/Thermal/Thermal Elements/Radiative Heat Transfer  area=ingenuityParams.battery.thermal.radToBox.area m^2  rad_tr_coeff=ingenuityParams.battery.thermal.radToBox.radCoeff W/(m^2*K^4)  T_specify=off  T_priority=None  T=0 K  T_nominal_specify=off  T_nominal_unit=K  T_nominal_value=1  Q_specify=off  Q_priority=None  Q=0 W  Q_nominal_specify=off  Q_nominal_unit=W  Q_nominal_value=1
      settings: SourceProductBaseCode=PW,SS,VE  LogSimulationData=on  InternalSimscapePortConfiguration="{\"Bottom\":[],\"Left\":[{\"id\":\"A\",\"label\":\"A\",\"type\":\"foundation.thermal.thermal\"}],\"Right\":[{\"id\":\"B\",\"label\":\"B\",\"type\":\"foundation.thermal.thermal\"}],\"Top\":[]}"
  RadiationToEnvironment : fl_lib/Thermal/Thermal Elements/Radiative Heat Transfer  area=ingenuityParams.battery.thermal.radToEnvironment.area m^2  rad_tr_coeff=ingenuityParams.battery.thermal.radToEnvironment.radCoeff W/(m^2*K^4)  T_specify=off  T_priority=None  T=0 K  T_nominal_specify=off  T_nominal_unit=K  T_nominal_value=1  Q_specify=off  Q_priority=None  Q=0 W  Q_nominal_specify=off  Q_nominal_unit=W  Q_nominal_value=1
      settings: SourceProductBaseCode=PW,SS,VE  LogSimulationData=on  InternalSimscapePortConfiguration="{\"Bottom\":[],\"Left\":[{\"id\":\"A\",\"label\":\"A\",\"type\":\"foundation.thermal.thermal\"}],\"Right\":[{\"id\":\"B\",\"label\":\"B\",\"type\":\"foundation.thermal.thermal\"}],\"Top\":[]}"
  SocSensor : TransferFcn  Denominator=[1 1]
  TempSensor : TransferFcn  Denominator=[1 1]
  Temperature Sensor : fl_lib/Thermal/Thermal Sensors/Temperature Sensor
      settings: SourceProductBaseCode=PW,SS,VE  LogSimulationData=on
  Thermal Reference : fl_lib/Thermal/Thermal Elements/Thermal Reference
      settings: SourceProductBaseCode=PW,SS,VE
  + : PMIOPort  Side=Left
  HEAT : PMIOPort  Port=2  Side=Right
  ENV : PMIOPort  Port=3  Side=Right
  - : PMIOPort  Port=4  Side=Right
  Bus Element Out : Outport  PortName=battery  Element=SOC3
  Bus Element Out1 : Outport  PortName=battery  Element=T3
  wires:
  SocSensor/1 -> Bus Element Out/1
  PS-Simulink Converter1/1 -> TempSensor/1
  PS-Simulink Converter3/1 -> SocSensor/1
  TempSensor/1 -> Bus Element Out1/1
  connections:
  Rad2box3/RConn1 -- Rad2box2/RConn1 -- Rad2box1/RConn1 -- Rad2box4/RConn1 -- Rad2box6/RConn1 -- Rad2box5/RConn1 -- InsulationLayer/LConn1 -- InsulantThermalMass/LConn1
  Cell2cellCond23/LConn1 -- Cell2/RConn2 -- Cell2cellCond12/RConn1 -- Rad2box2/LConn1
  Rad2box1/LConn1 -- Cell1/RConn2 -- Cell2cellCond12/LConn1
  Cell2cellCond34/RConn1 -- Cell2cellCond45/LConn1 -- Cell4/RConn2 -- Rad2box4/LConn1
  Cell2cellCond56/RConn1 -- Cell6/RConn2 -- Rad2box6/LConn1
  Cell2cellCond56/LConn1 -- Cell5/RConn2 -- Cell2cellCond45/RConn1 -- Rad2box5/LConn1
  Cell2cellCond23/RConn1 -- Rad2box3/LConn1 -- Cell2cellCond34/LConn1 -- Temperature Sensor/LConn1 -- Cell3/RConn2 -- HEAT/RConn1
  Cell3/LConn2 -- PS-Simulink Converter3/LConn1
  Cell2/LConn1 -- Cell3/RConn1
  RadiationToEnvironment/LConn1 -- InsulationLayer/RConn1
  ENV/RConn1 -- RadiationToEnvironment/RConn1
  Cell6/RConn1 -- Cell5/LConn1
  Cell2/RConn1 -- Cell1/LConn1
  Cell6/LConn1 -- +/RConn1
  Thermal Reference/LConn1 -- Temperature Sensor/RConn1
  Cell5/RConn1 -- Cell4/LConn1
  Cell4/RConn1 -- Cell3/LConn1
  Temperature Sensor/RConn2 -- PS-Simulink Converter1/LConn1
  -/RConn1 -- Cell1/RConn1

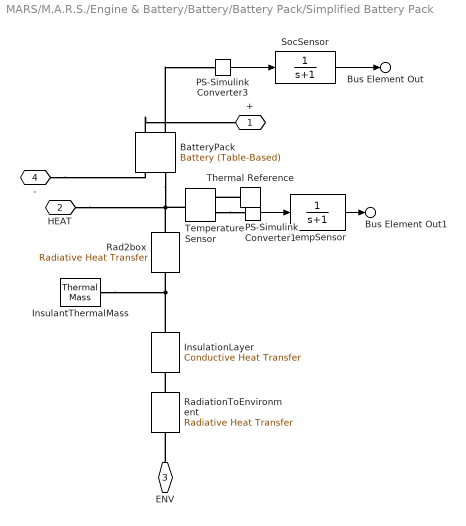
== system MARS/M.A.R.S./Engine & Battery/Battery/Battery Pack/Simplified Battery Pack ==
  BatteryPack : ee_lib/Sources/Battery (Table-Based)  SOC_vec=ingenuityParams.battery.cell.SOCvec  T_dependence=ee.enum.temperature_dependence.yes  prm_dir=ee.enum.battery.prm_dir.noCurrentDirectionality  T_vec=ingenuityParams.battery.cell.Tvec degC  V0_mat=ingenuityParams.battery.cell.V0_TLU*ingenuityParams.battery.numSeriesCells V  V0_vec=[3.1, 3.27, 3.31, 3.5] V  R0_mat=ingenuityParams.battery.cell.R0_TLU*ingenuityParams.battery.numSeriesCells/ingenuityParams.battery.numParallelStrings Ohm  R0_vec=[.015, .017, .012, .013] Ohm  R0_dis_mat=[.03, .015, .002; .04, .017, .008; .039, .012, .006; .027, .013, .021] Ohm  R0_dis_vec=[.015, .017, .012, .013] Ohm  R0_ch_mat=[.03, .015, .002; .04, .017, .008; .039, .012, .006; .027, .013, .021] Ohm  R0_ch_vec=[.015, .017, .012, .013] Ohm  AH=ingenuityParams.battery.cell.AH_TLU*ingenuityParams.battery.numParallelStrings A*hr  prm_leak=ee.enum.battery.prm_leak.disabled  Rleak_vec=[8000, 7000, 6000] Ohm  Rleak=7e3 Ohm  extrapolation_option=simscape.enum.extrapolation.nearest  SOC_port=ee.enum.enable.yes  V_range=[0, inf] V  prm_dyn=ee.enum.battery.prm_dyn.off  R1_mat=[.089, .076, .01; .042, .022, .099; .019, .007, .002; .051, .043, .029] Ohm  R1_vec=[.076, .022, .007, .043] Ohm  tau1_mat=[44, 148, 235; 93, 110, 1000; 19, 27, 133; .5, 22, 3] s  tau1_vec=[148, 110, 27, 22] s  R2_mat=[.014, .382, .407; .028, .006, .007; .014, .007, .006; .333, .956, .912] Ohm  R2_vec=[.382, .006, .007, .956] Ohm  tau2_mat=[1, 44, 5644; 11, 24, 506; 2, 14, 330; 3310, 13419, 30216] s  tau2_vec=[44, 24, 14, 13419] s  R3_mat=[.014, .382, .407; .028, .006, .007; .014, .007, .006; .333, .956, .912] Ohm  R3_vec=[.382, .006, .007, .956] Ohm  tau3_mat=[1, 44, 5644; 11, 24, 506; 2, 14, 330; 3310, 13419, 30216] s  tau3_vec=[44, 24, 14, 13419] s  R4_mat=[.014, .382, .407; .028, .006, .007; .014, .007, .006; .333, .956, .912] Ohm  R4_vec=[.382, .006, .007, .956] Ohm  tau4_mat=[1, 44, 5644; 11, 24, 506; 2, 14, 330; 3310, 13419, 30216] s  tau4_vec=[44, 24, 14, 13419] s  R5_mat=[.014, .382, .407; .028, .006, .007; .014, .007, .006; .333, .956, .912] Ohm  R5_vec=[.382, .006, .007, .956] Ohm  tau5_mat=[1, 44, 5644; 11, 24, 506; 2, 14, 330; 3310, 13419, 30216] s  tau5_vec=[44, 24, 14, 13419] s  prm_fade=ee.enum.battery.prm_fade.equations  N0=100  dV0=0  dR0=0  dAH=0  dRleak=0  dR1=0  dR2=0  dR3=0  dR4=0  dR5=0  N0vec=[100, 200, 300]  Tfadevec=[298.15, 323.15] K  dV0vec=[0, 0, 0]  dR0vec=[0, 0, 0]  dAHvec=[0, 0, 0]  dRleakvec=[0, 0, 0]  dR1vec=[0, 0, 0]  dR2vec=[0, 0, 0]  dR3vec=[0, 0, 0]  dR4vec=[0, 0, 0]  dR5vec=[0, 0, 0]  dV0mat=[0, 0; 0, 0; 0, 0]  dR0mat=[0, 0; 0, 0; 0, 0]  dAHmat=[0, 0; 0, 0; 0, 0]  dRleakmat=[0, 0; 0, 0; 0, 0]  dR1mat=[0, 0; 0, 0; 0, 0]  dR2mat=[0, 0; 0, 0; 0, 0]  dR3mat=[0, 0; 0, 0; 0, 0]  dR4mat=[0, 0; 0, 0; 0, 0]  dR5mat=[0, 0; 0, 0; 0, 0]  prm_age_modeling=ee.enum.battery.prm_age_modeling.equation  storage_dt_age_vec=[0] d  storage_T_age_vec=[273] K  prm_age_OCV=ee.enum.battery.prm_age_OCV.OCV  OCV_age=0.9  SOC_age=0.6  prm_age_resistance=ee.enum.battery.prm_age.disabled  OCV_scaling_age_resistance=2.2134e6  OCV_offset_age_resistance=1.632e6  temp_exp_age_resistance=0.515833569 V  t_exp_age_resistance=0.75  T_age_vec_resistance=[273.15, 298.15, 323.15] K  dt_age_vec_resistance=[90, 180, 270, 360] d  dR0_age_vec=[0, 0, 0]  t_meas_dR0_age=100 d  dR0_age_mat=[0, 0, 0; 0, 0, 0; 0, 0, 0; 0, 0, 0]  prm_age_capacity=ee.enum.battery.prm_age.disabled  OCV_scaling_age_capacity=1.5097e07  OCV_offset_age_capacity=8.3625e06  temp_exp_age_capacity=0.6011 V  t_exp_age_capacity=0.75  T_age_vec_capacity=[273.15, 298.15, 323.15] K  dt_age_vec_capacity=[90, 180, 270, 360] d  dAH_age_vec=[0, 0, 0]  t_meas_dAH_age=100 d  dAH_age_mat=[0, 0, 0; 0, 0, 0; 0, 0, 0; 0, 0, 0]  thermal_port=simscape.enum.thermaleffects.model  temperature=ingenuityParams.battery.cell.T_init degC  thermal_mass=ingenuityParams.battery.cell.mass*ingenuityParams.battery.cell.cp*ingenuityParams.battery.numCells J/K  i_specify=off  i_priority=None  i=0 A  i_nominal_specify=off  i_nominal_unit=A  i_nominal_value=1  v_specify=off  v_priority=None  v=0 V  v_nominal_specify=off  v_nominal_unit=V  v_nominal_value=1  stateOfCharge_specify=on  stateOfCharge_priority=High  stateOfCharge=ingenuityParams.battery.cell.SOC_init  stateOfCharge_nominal_specify=off  stateOfCharge_nominal_unit=1  stateOfCharge_nominal_value=1  num_cycles_specify=off  num_cycles_priority=High  num_cycles=0  num_cycles_nominal_specify=off  num_cycles_nominal_unit=1  num_cycles_nominal_value=1  cell_temperature_specify=on  cell_temperature_priority=High  cell_temperature=ingenuityParams.battery.cell.T_init degC  cell_temperature_nominal_specify=off  cell_temperature_nominal_unit=K  cell_temperature_nominal_value=1
      settings: SourceProductBaseCode=PS  LogSimulationData=on  InternalSimscapePortConfiguration="{\"Bottom\":[],\"Left\":[{\"id\":\"p\",\"label\":\"+\",\"type\":\"foundation.electrical.electrical\"},{\"id\":\"soc\",\"label\":\"SOC\",\"type\":\"output\"}],\"Right\":[{\"id\":\"n\",\"label\":\"-\",\"type\":\"foundation.electrical.electrical\"},{\"id\":\"H\",\"label\":\"H\",\"type\":\"foundation.thermal.thermal\"}],\"Top\":[]}"
  InsulantThermalMass : fl_lib/Thermal/Thermal Elements/Thermal Mass  mass=ingenuityParams.battery.thermal.insulantThermalMass.mass kg  sp_heat=ingenuityParams.battery.thermal.insulantThermalMass.cp J/kg/K  T_specify=on  T_priority=High  T=ingenuityParams.battery.cell.T_init degC  T_nominal_specify=off  T_nominal_unit=K  T_nominal_value=1  Q_specify=off  Q_priority=None  Q=0 W  Q_nominal_specify=off  Q_nominal_unit=W  Q_nominal_value=1
      settings: SourceProductBaseCode=PW,SS,VE  LogSimulationData=on
  InsulationLayer : fl_lib/Thermal/Thermal Elements/Conductive Heat Transfer  area=ingenuityParams.battery.thermal.insulationLayer.area m^2  thickness=ingenuityParams.battery.thermal.insulationLayer.thick m  th_cond=ingenuityParams.battery.thermal.insulationLayer.k W/(m*K)  T_specify=off  T_priority=None  T=0 K  T_nominal_specify=off  T_nominal_unit=K  T_nominal_value=1  Q_specify=off  Q_priority=None  Q=0 W  Q_nominal_specify=off  Q_nominal_unit=W  Q_nominal_value=1
      settings: SourceProductBaseCode=PW,SS,VE  LogSimulationData=on
  PS-Simulink Converter1 : nesl_utility/PS-Simulink Converter  PhysicalDomain=network_engine_domain  SubClassName=ps_output  LeftPortType=input  RightPortType=output  PseudoPeriodic=off  Frequencies=[]  VectorFormat=1-D array  Unit=degC  AffineConversion=on
      settings: SourceProductBaseCode=SS,PW,VE
  PS-Simulink Converter3 : nesl_utility/PS-Simulink Converter  PhysicalDomain=network_engine_domain  SubClassName=ps_output  LeftPortType=input  RightPortType=output  PseudoPeriodic=off  Frequencies=[]  VectorFormat=1-D array  Unit=1  AffineConversion=off
      settings: SourceProductBaseCode=SS,PW,VE
  Rad2box : fl_lib/Thermal/Thermal Elements/Radiative Heat Transfer  area=ingenuityParams.battery.thermal.radToBox.area*ingenuityParams.battery.numCells m^2  rad_tr_coeff=ingenuityParams.battery.thermal.radToBox.radCoeff W/(m^2*K^4)  T_specify=off  T_priority=None  T=0 K  T_nominal_specify=off  T_nominal_unit=K  T_nominal_value=1  Q_specify=off  Q_priority=None  Q=0 W  Q_nominal_specify=off  Q_nominal_unit=W  Q_nominal_value=1
      settings: SourceProductBaseCode=PW,SS,VE  LogSimulationData=on  InternalSimscapePortConfiguration="{\"Bottom\":[],\"Left\":[{\"id\":\"A\",\"label\":\"A\",\"type\":\"foundation.thermal.thermal\"}],\"Right\":[{\"id\":\"B\",\"label\":\"B\",\"type\":\"foundation.thermal.thermal\"}],\"Top\":[]}"
  RadiationToEnvironment : fl_lib/Thermal/Thermal Elements/Radiative Heat Transfer  area=ingenuityParams.battery.thermal.radToEnvironment.area m^2  rad_tr_coeff=ingenuityParams.battery.thermal.radToEnvironment.radCoeff W/(m^2*K^4)  T_specify=off  T_priority=None  T=0 K  T_nominal_specify=off  T_nominal_unit=K  T_nominal_value=1  Q_specify=off  Q_priority=None  Q=0 W  Q_nominal_specify=off  Q_nominal_unit=W  Q_nominal_value=1
      settings: SourceProductBaseCode=PW,SS,VE  LogSimulationData=on  InternalSimscapePortConfiguration="{\"Bottom\":[],\"Left\":[{\"id\":\"A\",\"label\":\"A\",\"type\":\"foundation.thermal.thermal\"}],\"Right\":[{\"id\":\"B\",\"label\":\"B\",\"type\":\"foundation.thermal.thermal\"}],\"Top\":[]}"
  SocSensor : TransferFcn  Denominator=[1 1]
  TempSensor : TransferFcn  Denominator=[1 1]
  Temperature Sensor : fl_lib/Thermal/Thermal Sensors/Temperature Sensor
      settings: SourceProductBaseCode=PW,SS,VE  LogSimulationData=on
  Thermal Reference : fl_lib/Thermal/Thermal Elements/Thermal Reference
      settings: SourceProductBaseCode=PW,SS,VE
  + : PMIOPort  Side=Left
  HEAT : PMIOPort  Port=2  Side=Right
  ENV : PMIOPort  Port=3  Side=Right
  - : PMIOPort  Port=4  Side=Right
  Bus Element Out : Outport  PortName=battery  Element=SOC3
  Bus Element Out1 : Outport  PortName=battery  Element=T3
  wires:
  SocSensor/1 -> Bus Element Out/1
  PS-Simulink Converter1/1 -> TempSensor/1
  PS-Simulink Converter3/1 -> SocSensor/1
  TempSensor/1 -> Bus Element Out1/1
  connections:
  InsulationLayer/LConn1 -- InsulantThermalMass/LConn1 -- Rad2box/RConn1
  BatteryPack/RConn2 -- Rad2box/LConn1 -- Temperature Sensor/LConn1 -- HEAT/RConn1
  BatteryPack/LConn2 -- PS-Simulink Converter3/LConn1
  RadiationToEnvironment/LConn1 -- InsulationLayer/RConn1
  ENV/RConn1 -- RadiationToEnvironment/RConn1
  BatteryPack/LConn1 -- +/RConn1
  Thermal Reference/LConn1 -- Temperature Sensor/RConn1
  Temperature Sensor/RConn2 -- PS-Simulink Converter1/LConn1
  -/RConn1 -- BatteryPack/RConn1
